simulink model "mainV02"  (R2016b)
settings: Solver=ode45  StartTime=0.0  StopTime=2000  MaxStep=0.2  RelTol=1e-2
undefined symbols (not defined in the file): checks, delta_e, deltae_degrees, deltat_1, deltat_2, deltat_3, deltat_4, deltat_5, Earth, ft, initialValues, LD, m, Newton, Raphson, s, WGS84
libraries: aerolibutil x7, aerolibasang x5, simulink x5, aerolibbdyn x3, aerolibconvert2 x3, aerolibconvert x2, aerolibatmos2 x1, aerolibobsolete x1, aerolibadyn x1, aerolib6dof2 x1, aerolibtransform2 x1, vrlib x1
(part 3 of 3)

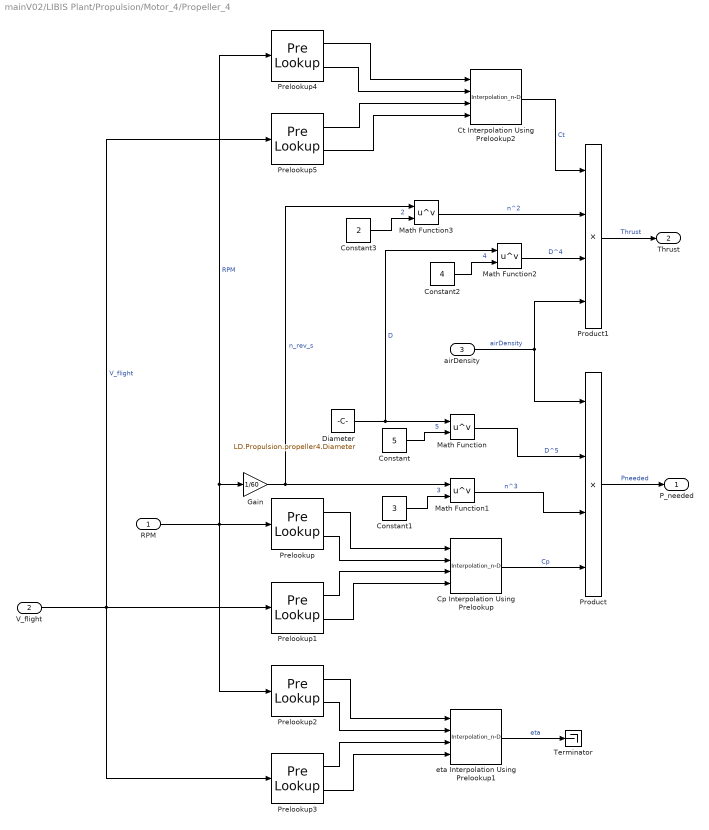
== system mainV02/LIBIS Plant/Propulsion/Motor_4/Propeller_4 ==
  RPM : Inport
  V_flight : Inport  Port=2
  airDensity : Inport  Port=3
  Constant : Constant  Value=5
  Constant1 : Constant  Value=3
  Constant2 : Constant  Value=4
  Constant3 : Constant  Value=2
  Cp Interpolation Using Prelookup : Interpolation_n-D  Table=LD.Propulsion.propeller4.Cp  InternalRulePriority=Speed
  Ct Interpolation Using Prelookup2 : Interpolation_n-D  Table=LD.Propulsion.propeller4.Ct  InternalRulePriority=Speed
  Diameter : Constant  Value=LD.Propulsion.propeller4.Diameter
  Gain : Gain  Gain=1/60
  Math Function{,1..3} (4 alike) : Math  Operator=pow  SaturateOnIntegerOverflow=on
  Prelookup : PreLookup  BreakpointsData=LD.Propulsion.propeller4.RPM  ExtrapMethod=Linear
  Prelookup1 : PreLookup  BreakpointsData=LD.Propulsion.propeller4.V  ExtrapMethod=Linear
  Prelookup2 : PreLookup  BreakpointsData=LD.Propulsion.propeller4.RPM  ExtrapMethod=Linear
  Prelookup3 : PreLookup  BreakpointsData=LD.Propulsion.propeller4.V  ExtrapMethod=Linear
  Prelookup4 : PreLookup  BreakpointsData=LD.Propulsion.propeller4.RPM  ExtrapMethod=Linear
  Prelookup5 : PreLookup  BreakpointsData=LD.Propulsion.propeller4.V  ExtrapMethod=Linear
  Product : Product  Inputs=4
  Product1 : Product  Inputs=4
  Terminator : Terminator
  eta Interpolation Using Prelookup1 : Interpolation_n-D  Table=LD.Propulsion.propeller4.eta  InternalRulePriority=Speed
  P_needed : Outport
  Thrust : Outport  Port=2
  wires:
  Prelookup/1 -> Cp Interpolation Using Prelookup/1
  Prelookup/2 -> Cp Interpolation Using Prelookup/2
  Prelookup1/1 -> Cp Interpolation Using Prelookup/3
  Prelookup1/2 -> Cp Interpolation Using Prelookup/4
  Diameter/1 -> Math Function2/1, Math Function/1  "D"
  Constant/1 -> Math Function/2  "5"
  Constant1/1 -> Math Function1/2  "3"
  Cp Interpolation Using Prelookup/1 -> Product/4  "Cp"
  Math Function1/1 -> Product/3  "n^3"
  Math Function/1 -> Product/2  "D^5"
  airDensity/1 -> Product/1, Product1/4  "airDensity"
  Product/1 -> P_needed/1  "Pneeded"
  Prelookup2/1 -> eta Interpolation Using Prelookup1/1
  Prelookup2/2 -> eta Interpolation Using Prelookup1/2
  Prelookup3/1 -> eta Interpolation Using Prelookup1/3
  Prelookup3/2 -> eta Interpolation Using Prelookup1/4
  Product1/1 -> Thrust/1  "Thrust"
  eta Interpolation Using Prelookup1/1 -> Terminator/1  "eta"
  RPM/1 -> Prelookup4/1, Gain/1, Prelookup/1, Prelookup2/1  "RPM"
  V_flight/1 -> Prelookup1/1, Prelookup5/1, Prelookup3/1  "V_flight"
  Constant2/1 -> Math Function2/2  "4"
  Math Function2/1 -> Product1/3  "D^4"
  Prelookup4/1 -> Ct Interpolation Using Prelookup2/1
  Prelookup4/2 -> Ct Interpolation Using Prelookup2/2
  Prelookup5/1 -> Ct Interpolation Using Prelookup2/3
  Prelookup5/2 -> Ct Interpolation Using Prelookup2/4
  Ct Interpolation Using Prelookup2/1 -> Product1/1  "Ct"
  Constant3/1 -> Math Function3/2  "2"
  Gain/1 -> Math Function3/1, Math Function1/1  "n_rev_s"
  Math Function3/1 -> Product1/2  "n^2"

== system mainV02/LIBIS Plant/Propulsion/Motor_5/ESC_5 ==
  V_battery : Inport  Unit=V
  Throttle : Inport  Port=2  Unit=1
  Constant : Constant
  Constant1 : Constant  Value=0
  Product : Product
  Product1 : Product
  Switch : Switch  Criteria=u2 > Threshold
  eta_ESC : Constant  Value=LD.Propulsion.ESC5.eta
  V_ESC : Outport  Unit=V
  isActiveMotor : Outport  Port=2
  wires:
  eta_ESC/1 -> Product/2
  V_battery/1 -> Product/1
  Product/1 -> Product1/1
  Product1/1 -> V_ESC/1
  Throttle/1 -> Product1/2, Switch/2
  Switch/1 -> isActiveMotor/1
  Constant/1 -> Switch/1
  Constant1/1 -> Switch/3

== system mainV02/LIBIS Plant/Propulsion/Motor_5/Motor_5 ==
  V_ESC : Inport
  isActive : Inport  Port=2
  Im : Inport  Port=3
  ActiveMotor5 : Subsystem  VariantControl=Variants.Motor2~=0
  Peje Switch : Switch  Criteria=u2 > Threshold
  RPM Switch : Switch  Criteria=u2 > Threshold
  noActiveMotor5 : Subsystem  VariantControl=Variants.Motor2==0
  RPM : Outport
  Peje : Outport  Port=2
  wires:
  V_ESC/1 -> noActiveMotor5/1(V_ESC), ActiveMotor5/1(V_ESC)
  Im/1 -> noActiveMotor5/2(Im), ActiveMotor5/2(Im)
  isActive/1 -> RPM Switch/2, Peje Switch/2
  Peje Switch/1 -> Peje/1
  RPM Switch/1 -> RPM/1
  ActiveMotor5/1(RPM) -> RPM Switch/1
  noActiveMotor5/1(RPM) -> RPM Switch/3
  noActiveMotor5/2(Peje) -> Peje Switch/3
  ActiveMotor5/2(Peje) -> Peje Switch/1

== system mainV02/LIBIS Plant/Propulsion/Motor_5/Propeller_5 ==
  RPM : Inport
  V_flight : Inport  Port=2
  airDensity : Inport  Port=3
  Constant : Constant  Value=5
  Constant1 : Constant  Value=3
  Constant2 : Constant  Value=4
  Constant3 : Constant  Value=2
  Cp Interpolation Using Prelookup : Interpolation_n-D  Table=LD.Propulsion.propeller5.Cp  InternalRulePriority=Speed
  Ct Interpolation Using Prelookup2 : Interpolation_n-D  Table=LD.Propulsion.propeller5.Ct  InternalRulePriority=Speed
  Diameter : Constant  Value=LD.Propulsion.propeller5.Diameter
  Gain : Gain  Gain=1/60
  Math Function{,1..3} (4 alike) : Math  Operator=pow  SaturateOnIntegerOverflow=on
  Prelookup : PreLookup  BreakpointsData=LD.Propulsion.propeller5.RPM  ExtrapMethod=Linear
  Prelookup1 : PreLookup  BreakpointsData=LD.Propulsion.propeller5.V  ExtrapMethod=Linear
  Prelookup2 : PreLookup  BreakpointsData=LD.Propulsion.propeller5.RPM  ExtrapMethod=Linear
  Prelookup3 : PreLookup  BreakpointsData=LD.Propulsion.propeller5.V  ExtrapMethod=Linear
  Prelookup4 : PreLookup  BreakpointsData=LD.Propulsion.propeller5.RPM  ExtrapMethod=Linear
  Prelookup5 : PreLookup  BreakpointsData=LD.Propulsion.propeller5.V  ExtrapMethod=Linear
  Product : Product  Inputs=4
  Product1 : Product  Inputs=4
  Terminator : Terminator
  eta Interpolation Using Prelookup1 : Interpolation_n-D  Table=LD.Propulsion.propeller5.eta  InternalRulePriority=Speed
  P_needed : Outport
  Thrust : Outport  Port=2
  wires:
  Prelookup/1 -> Cp Interpolation Using Prelookup/1
  Prelookup/2 -> Cp Interpolation Using Prelookup/2
  Prelookup1/1 -> Cp Interpolation Using Prelookup/3
  Prelookup1/2 -> Cp Interpolation Using Prelookup/4
  Diameter/1 -> Math Function2/1, Math Function/1  "D"
  Constant/1 -> Math Function/2  "5"
  Constant1/1 -> Math Function1/2  "3"
  Cp Interpolation Using Prelookup/1 -> Product/4  "Cp"
  Math Function1/1 -> Product/3  "n^3"
  Math Function/1 -> Product/2  "D^5"
  airDensity/1 -> Product/1, Product1/4  "airDensity"
  Product/1 -> P_needed/1  "Pneeded"
  Prelookup2/1 -> eta Interpolation Using Prelookup1/1
  Prelookup2/2 -> eta Interpolation Using Prelookup1/2
  Prelookup3/1 -> eta Interpolation Using Prelookup1/3
  Prelookup3/2 -> eta Interpolation Using Prelookup1/4
  Product1/1 -> Thrust/1  "Thrust"
  eta Interpolation Using Prelookup1/1 -> Terminator/1  "eta"
  RPM/1 -> Prelookup4/1, Gain/1, Prelookup/1, Prelookup2/1  "RPM"
  V_flight/1 -> Prelookup1/1, Prelookup5/1, Prelookup3/1  "V_flight"
  Constant2/1 -> Math Function2/2  "4"
  Math Function2/1 -> Product1/3  "D^4"
  Prelookup4/1 -> Ct Interpolation Using Prelookup2/1
  Prelookup4/2 -> Ct Interpolation Using Prelookup2/2
  Prelookup5/1 -> Ct Interpolation Using Prelookup2/3
  Prelookup5/2 -> Ct Interpolation Using Prelookup2/4
  Ct Interpolation Using Prelookup2/1 -> Product1/1  "Ct"
  Constant3/1 -> Math Function3/2  "2"
  Gain/1 -> Math Function3/1, Math Function1/1  "n_rev_s"
  Math Function3/1 -> Product1/2  "n^2"

== system mainV02/LIBIS Plant/Propulsion/Motor_1/Motor_1/ActiveMotor1 ==
  V_ESC : Inport
  Im : Inport  Port=2
  Display : Display
  Divide : Product  Inputs=*/*
  Divide1 : Product  Inputs=**
  Divide2 : Product  Inputs=/*
  I0 : Constant  Value=LD.Propulsion.motor1.I0
  Kv : Constant  Value=LD.Propulsion.motor1.Kv
  Product : Product
  Product1 : Product
  Rm : Constant  Value=LD.Propulsion.motor1.Rm
  Sum : Sum  Inputs=+-
  Sum1 : Sum  Inputs=+-
  RPM : Outport
  Peje : Outport  Port=2
  wires:
  I0/1 -> Sum1/2  "I0"
  Divide1/1 -> Divide2/1  "P_in"
  V_ESC/1 -> Divide1/1, Sum/1
  Sum/1 -> Product/1  "Vm - Rm·Im"
  Im/1 -> Sum1/1, Divide1/2, Product1/1
  Divide/1 -> Peje/1, Divide2/2  "Peje"
  Kv/1 -> Divide/2, Product/2  "Kv"
  Product/1 -> RPM/1, Divide/1  "RPM"
  Rm/1 -> Product1/2  "Rm"
  Product1/1 -> Sum/2  "Rm·Im"
  Divide2/1 -> Display/1  "eta_motor"
  Sum1/1 -> Divide/3  "Im-I0"

== system mainV02/LIBIS Plant/Propulsion/Motor_1/Motor_1/noActiveMotor1 ==
  V_ESC : Inport
  Im : Inport  Port=2
  Constant : Constant  Value=0
  Constant1 : Constant  Value=0
  Terminator : Terminator
  Terminator1 : Terminator
  RPM : Outport
  Peje : Outport  Port=2
  wires:
  V_ESC/1 -> Terminator/1
  Im/1 -> Terminator1/1
  Constant/1 -> RPM/1
  Constant1/1 -> Peje/1

== system mainV02/LIBIS Plant/Propulsion/Motor_2/Motor_2/ActiveMotor2 ==
  V_ESC : Inport
  Im : Inport  Port=2
  Display : Display
  Divide : Product  Inputs=*/*
  Divide1 : Product  Inputs=**
  Divide2 : Product  Inputs=/*
  I0 : Constant  Value=LD.Propulsion.motor2.I0
  Kv : Constant  Value=LD.Propulsion.motor2.Kv
  Product : Product
  Product1 : Product
  Rm : Constant  Value=LD.Propulsion.motor2.Rm
  Sum : Sum  Inputs=+-
  Sum1 : Sum  Inputs=+-
  RPM : Outport
  Peje : Outport  Port=2
  wires:
  I0/1 -> Sum1/2  "I0"
  Divide1/1 -> Divide2/1  "P_in"
  V_ESC/1 -> Divide1/1, Sum/1
  Sum/1 -> Product/1  "Vm - Rm·Im"
  Im/1 -> Sum1/1, Divide1/2, Product1/1
  Divide/1 -> Peje/1, Divide2/2  "Peje"
  Kv/1 -> Divide/2, Product/2  "Kv"
  Product/1 -> RPM/1, Divide/1  "RPM"
  Rm/1 -> Product1/2  "Rm"
  Product1/1 -> Sum/2  "Rm·Im"
  Divide2/1 -> Display/1  "eta_motor"
  Sum1/1 -> Divide/3  "Im-I0"

== system mainV02/LIBIS Plant/Propulsion/Motor_2/Motor_2/noActiveMotor2 ==
  V_ESC : Inport
  Im : Inport  Port=2
  Constant : Constant  Value=0
  Constant1 : Constant  Value=0
  Terminator : Terminator
  Terminator1 : Terminator
  RPM : Outport
  Peje : Outport  Port=2
  wires:
  V_ESC/1 -> Terminator/1
  Im/1 -> Terminator1/1
  Constant/1 -> RPM/1
  Constant1/1 -> Peje/1

== system mainV02/LIBIS Plant/Propulsion/Motor_3/Motor_3/ActiveMotor3 ==
  V_ESC : Inport
  Im : Inport  Port=2
  Display : Display
  Divide : Product  Inputs=*/*
  Divide1 : Product  Inputs=**
  Divide2 : Product  Inputs=/*
  I0 : Constant  Value=LD.Propulsion.motor3.I0
  Kv : Constant  Value=LD.Propulsion.motor3.Kv
  Product : Product
  Product1 : Product
  Rm : Constant  Value=LD.Propulsion.motor3.Rm
  Sum : Sum  Inputs=+-
  Sum1 : Sum  Inputs=+-
  RPM : Outport
  Peje : Outport  Port=2
  wires:
  I0/1 -> Sum1/2  "I0"
  Divide1/1 -> Divide2/1  "P_in"
  V_ESC/1 -> Divide1/1, Sum/1
  Sum/1 -> Product/1  "Vm - Rm·Im"
  Im/1 -> Sum1/1, Divide1/2, Product1/1
  Divide/1 -> Peje/1, Divide2/2  "Peje"
  Kv/1 -> Divide/2, Product/2  "Kv"
  Product/1 -> RPM/1, Divide/1  "RPM"
  Rm/1 -> Product1/2  "Rm"
  Product1/1 -> Sum/2  "Rm·Im"
  Divide2/1 -> Display/1  "eta_motor"
  Sum1/1 -> Divide/3  "Im-I0"

== system mainV02/LIBIS Plant/Propulsion/Motor_3/Motor_3/noActiveMotor3 ==
  V_ESC : Inport
  Im : Inport  Port=2
  Constant : Constant  Value=0
  Constant1 : Constant  Value=0
  Terminator : Terminator
  Terminator1 : Terminator
  RPM : Outport
  Peje : Outport  Port=2
  wires:
  V_ESC/1 -> Terminator/1
  Im/1 -> Terminator1/1
  Constant/1 -> RPM/1
  Constant1/1 -> Peje/1

== system mainV02/LIBIS Plant/Propulsion/Motor_4/Motor_4/ActiveMotor4 ==
  V_ESC : Inport
  Im : Inport  Port=2
  Display : Display
  Divide : Product  Inputs=*/*
  Divide1 : Product  Inputs=**
  Divide2 : Product  Inputs=/*
  I0 : Constant  Value=LD.Propulsion.motor4.I0
  Kv : Constant  Value=LD.Propulsion.motor4.Kv
  Product : Product
  Product1 : Product
  Rm : Constant  Value=LD.Propulsion.motor4.Rm
  Sum : Sum  Inputs=+-
  Sum1 : Sum  Inputs=+-
  RPM : Outport
  Peje : Outport  Port=2
  wires:
  I0/1 -> Sum1/2  "I0"
  Divide1/1 -> Divide2/1  "P_in"
  V_ESC/1 -> Divide1/1, Sum/1
  Sum/1 -> Product/1  "Vm - Rm·Im"
  Im/1 -> Sum1/1, Divide1/2, Product1/1
  Divide/1 -> Peje/1, Divide2/2  "Peje"
  Kv/1 -> Divide/2, Product/2  "Kv"
  Product/1 -> RPM/1, Divide/1  "RPM"
  Rm/1 -> Product1/2  "Rm"
  Product1/1 -> Sum/2  "Rm·Im"
  Divide2/1 -> Display/1  "eta_motor"
  Sum1/1 -> Divide/3  "Im-I0"

== system mainV02/LIBIS Plant/Propulsion/Motor_4/Motor_4/noActiveMotor4 ==
  V_ESC : Inport
  Im : Inport  Port=2
  Constant : Constant  Value=0
  Constant1 : Constant  Value=0
  Terminator : Terminator
  Terminator1 : Terminator
  RPM : Outport
  Peje : Outport  Port=2
  wires:
  V_ESC/1 -> Terminator/1
  Im/1 -> Terminator1/1
  Constant/1 -> RPM/1
  Constant1/1 -> Peje/1

== system mainV02/LIBIS Plant/Propulsion/Motor_5/Motor_5/ActiveMotor5 ==
  V_ESC : Inport
  Im : Inport  Port=2
  Display : Display
  Divide : Product  Inputs=*/*
  Divide1 : Product  Inputs=**
  Divide2 : Product  Inputs=/*
  I0 : Constant  Value=LD.Propulsion.motor5.I0
  Kv : Constant  Value=LD.Propulsion.motor5.Kv
  Product : Product
  Product1 : Product
  Rm : Constant  Value=LD.Propulsion.motor5.Rm
  Sum : Sum  Inputs=+-
  Sum1 : Sum  Inputs=+-
  RPM : Outport
  Peje : Outport  Port=2
  wires:
  I0/1 -> Sum1/2  "I0"
  Divide1/1 -> Divide2/1  "P_in"
  V_ESC/1 -> Divide1/1, Sum/1
  Sum/1 -> Product/1  "Vm - Rm·Im"
  Im/1 -> Sum1/1, Divide1/2, Product1/1
  Divide/1 -> Peje/1, Divide2/2  "Peje"
  Kv/1 -> Divide/2, Product/2  "Kv"
  Product/1 -> RPM/1, Divide/1  "RPM"
  Rm/1 -> Product1/2  "Rm"
  Product1/1 -> Sum/2  "Rm·Im"
  Divide2/1 -> Display/1  "eta_motor"
  Sum1/1 -> Divide/3  "Im-I0"

== system mainV02/LIBIS Plant/Propulsion/Motor_5/Motor_5/noActiveMotor5 ==
  V_ESC : Inport
  Im : Inport  Port=2
  Constant : Constant  Value=0
  Constant1 : Constant  Value=0
  Terminator : Terminator
  Terminator1 : Terminator
  RPM : Outport
  Peje : Outport  Port=2
  wires:
  V_ESC/1 -> Terminator/1
  Im/1 -> Terminator1/1
  Constant/1 -> RPM/1
  Constant1/1 -> Peje/1
